simulink model "NXT_circle"  (R2024b)
settings: Solver=FixedStepDiscrete  StartTime=0.0  StopTime=inf  FixedStep=Ts  RelTol=1e-3
values from neighbouring files (symbols this model uses):
  dt = 0.005    [main.m]    (also in make_smooth.m)
  joint1_pos_circle = [0 joint1_pos_circle]    [generate_circle_trajectory.m]
  joint2_pos_circle = [0 joint2_pos_circle]    [generate_circle_trajectory.m]
  joint3_pos_circle = [0]    [generate_circle_trajectory.m]
  Kd = 2    [main.m]
  Kp = 25    [main.m]
  motor1_vel_circle = [0 motor1_vel_circle]    [generate_circle_trajectory.m]
  motor2_vel_circle = [0 motor2_vel_circle]    [generate_circle_trajectory.m]
  motor3_vel_circle = [0 motor3_vel_circle]    [generate_circle_trajectory.m]
  Ts_traj = 0.1    [main.m]
libraries: legonxtlib x6, cstblocks x3
settings Model: SimulationMode=external  ExtModeTrigDuration=2  Creator=pwterry
settings SolverCC: AlgebraicLoopSolver=TrustRegion
settings DataIOCC: LimitDataPoints=on  SaveFormat=Array  ReturnWorkspaceOutputs=off
settings OptimizationCC: LifeSpan=1  EfficientTunableParamExpr=on
settings DebuggingCC: UnderspecifiedInitializationDetection=Classic  MergeDetectMultiDrivingBlocksExec=none  UnconnectedInputMsg=warning  UnconnectedOutputMsg=warning  UnconnectedLineMsg=warning  SFUnexpectedBacktrackingDiag=warning  SFNoUnconditionalDefaultTransitionDiag=warning  SFExecutionAtInitializationDiag=none  ArithmeticOperatorsInVariantConditions=warning
settings HardwareCC: ProdBitPerPointer=32  ProdBitPerSizeT=32  ProdBitPerPtrDiffT=32  ProdLargestAtomicInteger=Long  ProdIntDivRoundTo=Undefined  ProdWordSize=32  ProdHWDeviceType=ARM Compatible->ARM 7
settings ModelReferenceCC: PropagateSignalLabelsOutOfModel=off
settings SFSimCC: SimUseLocalCustomCode=off  MATLABDynamicMemAlloc=off  CustomCodeUndefinedFunction=UseInterfaceOnly
settings RTWCC: Description=Run on Target Hardware  SystemTargetFile=realtime.tlc  GenerateMakefile=off  TemplateMakefile=realtime.tmf  RTWVerbose=off  RTWUseLocalCustomCode=off  GPUComputeCapability=3.5
settings CodeAppCC: StateflowObjectComments=on
settings STFCustomTargetCC: TargetLibSuffix=.a  GenerateSampleERTMain=on  ERTCustomFileBanners=on  SupportNonInlinedSFcns=off  RemoveResetFunc=on  SupportVariableSizeSignals=on  MATLABClassNameForMDSCustomization=Simulink.SoftwareTarget.ERTCustomization  SystemTargetFile=realtime.tlc
settings ERTTargetCC: MultiwordLength=2048  GenerateSampleERTMain=on  ParMdlRefBuildCompliant=off  CompOptLevelCompliant=off  ConcurrentExecutionCompliant=off  CombineOutputUpdateFcns=off  SupportContinuousTime=on  SupportVariableSizeSignals=on  ModelStepFunctionPrototypeControlCompliant=off  CPPClassGenCompliant=off  UseToolchainInfoCompliant=off  ExtMode=on  ExtModeTransport=2  ExtModeMexArgs=0 233 9600 30  InlinedParameterPlacement=Hierarchical  ERTSrcFileBannerTemplate=realtime_code_template.cgt  ERTHdrFileBannerTemplate=realtime_code_template.cgt  ERTDataSrcFileTemplate=realtime_code_template.cgt  ERTDataHdrFileTemplate=realtime_code_template.cgt  ERTCustomFileTemplate=realtime_file_process.tlc  ConvertIfToSwitch=off  SuppressUnreachableDefaultCases=off  DynamicArrayContainerType=coder::array
settings ConfigComp: CovMetricSettings=dw  CovSaveCumulativeToWorkspaceVar=on  CovSaveSingleToWorkspaceVar=on  CovExternalEMLEnable=off  CovSFcnEnable=off

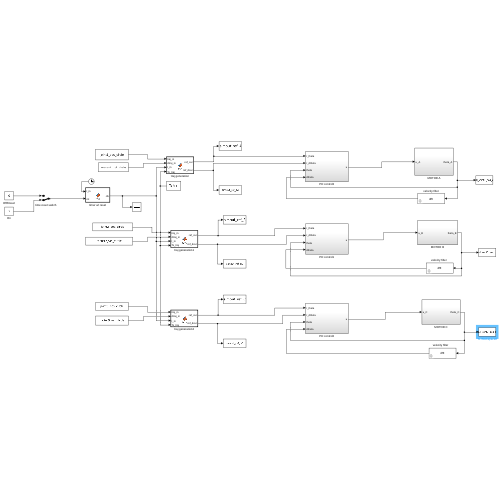
[thumbnail: Simulink's stored preview of the top-level diagram]
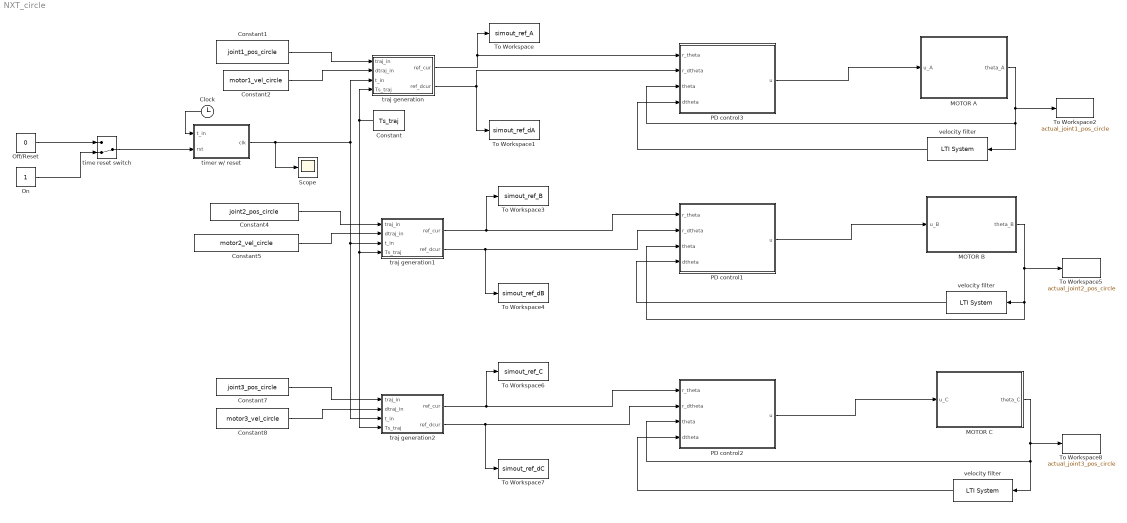
== system NXT_circle ==
  Clock : Clock
  Constant : Constant  Value=Ts_traj
  Constant1 : Constant  Value=joint1_pos_circle  SampleTime=dt
  Constant2 : Constant  Value=motor1_vel_circle  SampleTime=dt
  Constant4 : Constant  Value=joint2_pos_circle  SampleTime=dt
  Constant5 : Constant  Value=motor2_vel_circle  SampleTime=dt
  Constant7 : Constant  Value=joint3_pos_circle  SampleTime=dt
  Constant8 : Constant  Value=motor3_vel_circle  SampleTime=dt
  MOTOR A : Subsystem
  MOTOR B : Subsystem
  MOTOR C : Subsystem
  Off/Reset : Constant  Value=0
  On : Constant
  PD control1 : Subsystem
  PD control2 : Subsystem
  PD control3 : Subsystem
  Scope : Scope
  To Workspace : ToWorkspace  VariableName=simout_ref_A  SaveFormat=Structure With Time  SampleTime=-1
  To Workspace1 : ToWorkspace  VariableName=simout_ref_dA  SaveFormat=Structure With Time  SampleTime=-1
  To Workspace2 : ToWorkspace  VariableName=actual_joint1_pos_circle  SaveFormat=Structure With Time  SampleTime=dt
  To Workspace3 : ToWorkspace  VariableName=simout_ref_B  SaveFormat=Structure With Time  SampleTime=-1
  To Workspace4 : ToWorkspace  VariableName=simout_ref_dB  SaveFormat=Structure With Time  SampleTime=-1
  To Workspace5 : ToWorkspace  VariableName=actual_joint2_pos_circle  SaveFormat=Structure With Time  SampleTime=dt
  To Workspace6 : ToWorkspace  VariableName=simout_ref_C  SaveFormat=Structure With Time  SampleTime=-1
  To Workspace7 : ToWorkspace  VariableName=simout_ref_dC  SaveFormat=Structure With Time  SampleTime=-1
  To Workspace8 : ToWorkspace  VariableName=actual_joint3_pos_circle  SaveFormat=Structure With Time  SampleTime=dt
  time reset switch : ManualSwitch  CurrentSetting=0
  timer w/ reset : MATLAB Function  TreatAsAtomicUnit=on
  traj generation : MATLAB Function  TreatAsAtomicUnit=on
  traj generation1 : MATLAB Function  TreatAsAtomicUnit=on
  traj generation2 : MATLAB Function  TreatAsAtomicUnit=on
  velocity filter : cstblocks/LTI System  sys=dfft  IC=[]  PadeOrder=0
  "velocity filter  " : cstblocks/LTI System  sys=dfft  IC=[]  PadeOrder=0
  "velocity filter     " : cstblocks/LTI System  sys=dfft  IC=[]  PadeOrder=0
  wires:
  Constant/1 -> traj generation2/4(Ts_traj), traj generation1/4(Ts_traj), traj generation/4(Ts_traj)
  timer w/ reset/1(clk) -> Scope/1, traj generation1/3(t_in), traj generation2/3(t_in), traj generation/3(t_in)
  Constant1/1 -> traj generation/1(traj_in)
  Constant2/1 -> traj generation/2(dtraj_in)
  traj generation/1(ref_cur) -> PD control3/1(r_theta), To Workspace/1
  traj generation/2(ref_dcur) -> PD control3/2(r_dtheta), To Workspace1/1
  Constant4/1 -> traj generation1/1(traj_in)
  Constant5/1 -> traj generation1/2(dtraj_in)
  traj generation1/1(ref_cur) -> PD control1/1(r_theta), To Workspace3/1
  traj generation1/2(ref_dcur) -> PD control1/2(r_dtheta), To Workspace4/1
  Constant7/1 -> traj generation2/1(traj_in)
  Constant8/1 -> traj generation2/2(dtraj_in)
  traj generation2/1(ref_cur) -> PD control2/1(r_theta), To Workspace6/1
  traj generation2/2(ref_dcur) -> PD control2/2(r_dtheta), To Workspace7/1
  MOTOR A/1(theta_A) -> To Workspace2/1, PD control3/3(theta), velocity filter/1
  velocity filter/1 -> PD control3/4(dtheta)
  MOTOR B/1(theta_B) -> To Workspace5/1, PD control1/3(theta), "velocity filter  "/1
  "velocity filter  "/1 -> PD control1/4(dtheta)
  "velocity filter     "/1 -> PD control2/4(dtheta)
  MOTOR C/1(theta_C) -> To Workspace8/1, PD control2/3(theta), "velocity filter     "/1
  Off/Reset/1 -> time reset switch/1
  On/1 -> time reset switch/2
  time reset switch/1 -> timer w/ reset/2(rst)
  Clock/1 -> timer w/ reset/1(t_in)
  PD control3/1(u) -> MOTOR A/1(u_A)
  PD control1/1(u) -> MOTOR B/1(u_B)
  PD control2/1(u) -> MOTOR C/1(u_C)

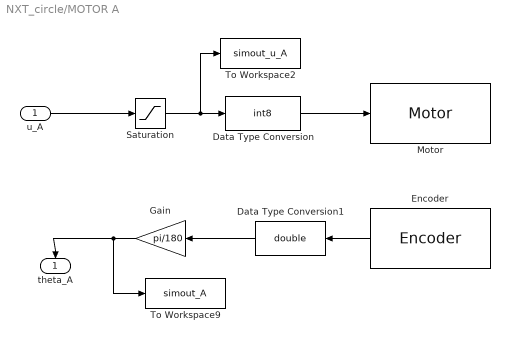
== system NXT_circle/MOTOR A ==
  u_A : Inport
  Data Type Conversion : DataTypeConversion  OutDataTypeStr=int8  SaturateOnIntegerOverflow=off  RndMeth=Floor
  Data Type Conversion1 : DataTypeConversion  OutDataTypeStr=double  SaturateOnIntegerOverflow=off  RndMeth=Floor
  Encoder : legonxtlib/Encoder  portNumber=A  opMode=No reset  sampleTime=Ts
  Gain : Gain  Gain=pi/180
  Motor : legonxtlib/Motor  sportNumber=A  sstopAction=Brake
  Saturation : Saturate  UpperLimit=100  LowerLimit=-100
  To Workspace2 : ToWorkspace  VariableName=simout_u_A  SaveFormat=Structure With Time  SampleTime=-1
  To Workspace9 : ToWorkspace  VariableName=simout_A  SaveFormat=Structure With Time  SampleTime=-1
  theta_A : Outport
  wires:
  u_A/1 -> Saturation/1
  Data Type Conversion1/1 -> Gain/1
  Saturation/1 -> To Workspace2/1, Data Type Conversion/1
  Encoder/1 -> Data Type Conversion1/1
  Data Type Conversion/1 -> Motor/1
  Gain/1 -> theta_A/1, To Workspace9/1

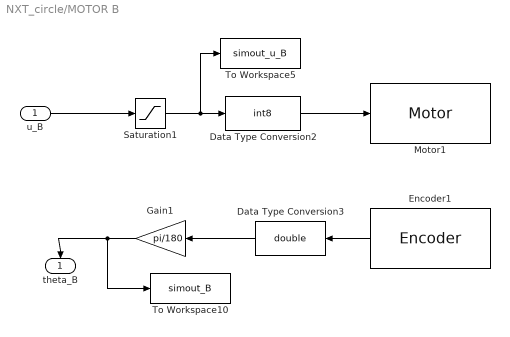
== system NXT_circle/MOTOR B ==
  u_B : Inport
  Data Type Conversion2 : DataTypeConversion  OutDataTypeStr=int8  SaturateOnIntegerOverflow=off  RndMeth=Floor
  Data Type Conversion3 : DataTypeConversion  OutDataTypeStr=double  SaturateOnIntegerOverflow=off  RndMeth=Floor
  Encoder1 : legonxtlib/Encoder  portNumber=B  opMode=No reset  sampleTime=Ts
  Gain1 : Gain  Gain=pi/180
  Motor1 : legonxtlib/Motor  sportNumber=B  sstopAction=Brake
  Saturation1 : Saturate  UpperLimit=100  LowerLimit=-100
  To Workspace10 : ToWorkspace  VariableName=simout_B  SaveFormat=Structure With Time  SampleTime=-1
  To Workspace5 : ToWorkspace  VariableName=simout_u_B  SaveFormat=Structure With Time  SampleTime=-1
  theta_B : Outport
  wires:
  Encoder1/1 -> Data Type Conversion3/1
  u_B/1 -> Saturation1/1
  Saturation1/1 -> To Workspace5/1, Data Type Conversion2/1
  Data Type Conversion3/1 -> Gain1/1
  Data Type Conversion2/1 -> Motor1/1
  Gain1/1 -> theta_B/1, To Workspace10/1

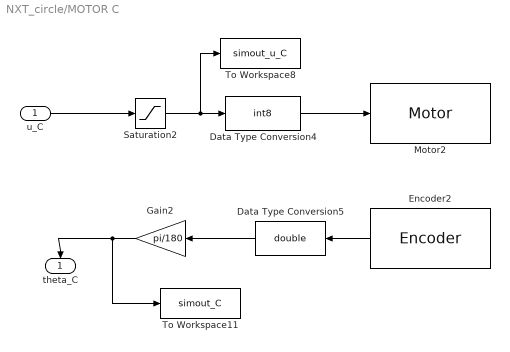
== system NXT_circle/MOTOR C ==
  u_C : Inport
  Data Type Conversion4 : DataTypeConversion  OutDataTypeStr=int8  SaturateOnIntegerOverflow=off  RndMeth=Floor
  Data Type Conversion5 : DataTypeConversion  OutDataTypeStr=double  SaturateOnIntegerOverflow=off  RndMeth=Floor
  Encoder2 : legonxtlib/Encoder  portNumber=C  opMode=No reset  sampleTime=Ts
  Gain2 : Gain  Gain=pi/180
  Motor2 : legonxtlib/Motor  sportNumber=C  sstopAction=Brake
  Saturation2 : Saturate  UpperLimit=100  LowerLimit=-100
  To Workspace11 : ToWorkspace  VariableName=simout_C  SaveFormat=Structure With Time  SampleTime=-1
  To Workspace8 : ToWorkspace  VariableName=simout_u_C  SaveFormat=Structure With Time  SampleTime=-1
  theta_C : Outport
  wires:
  Encoder2/1 -> Data Type Conversion5/1
  Data Type Conversion4/1 -> Motor2/1
  Data Type Conversion5/1 -> Gain2/1
  Gain2/1 -> theta_C/1, To Workspace11/1
  Saturation2/1 -> To Workspace8/1, Data Type Conversion4/1
  u_C/1 -> Saturation2/1

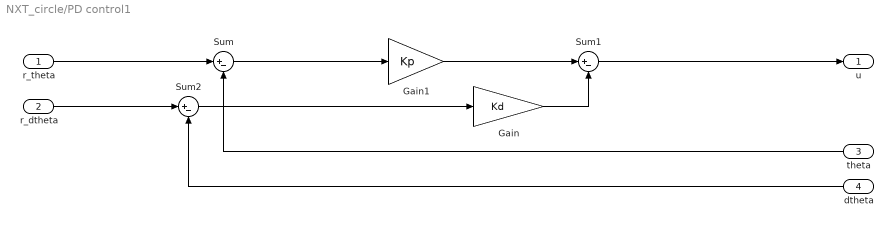
== system NXT_circle/PD control1 ==
  r_theta : Inport
  r_dtheta : Inport  Port=2
  theta : Inport  Port=3
  dtheta : Inport  Port=4
  Gain : Gain  Gain=Kd  SampleTime=dt
  Gain1 : Gain  Gain=Kp  SampleTime=dt
  Sum : Sum  Inputs=|+-
  Sum1 : Sum  Inputs=|+-
  Sum2 : Sum  Inputs=|+-
  u : Outport
  wires:
  r_theta/1 -> Sum/1
  Sum/1 -> Gain1/1
  theta/1 -> Sum/2
  dtheta/1 -> Sum2/2
  Gain1/1 -> Sum1/1
  Sum1/1 -> u/1
  r_dtheta/1 -> Sum2/1
  Sum2/1 -> Gain/1
  Gain/1 -> Sum1/2

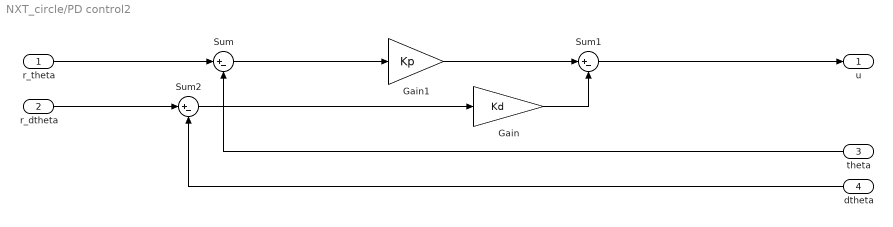
== system NXT_circle/PD control2 ==
  r_theta : Inport
  r_dtheta : Inport  Port=2
  theta : Inport  Port=3
  dtheta : Inport  Port=4
  Gain : Gain  Gain=Kd  SampleTime=dt
  Gain1 : Gain  Gain=Kp  SampleTime=dt
  Sum : Sum  Inputs=|+-
  Sum1 : Sum  Inputs=|+-
  Sum2 : Sum  Inputs=|+-
  u : Outport
  wires:
  r_theta/1 -> Sum/1
  Sum/1 -> Gain1/1
  theta/1 -> Sum/2
  dtheta/1 -> Sum2/2
  Gain1/1 -> Sum1/1
  Sum1/1 -> u/1
  r_dtheta/1 -> Sum2/1
  Sum2/1 -> Gain/1
  Gain/1 -> Sum1/2

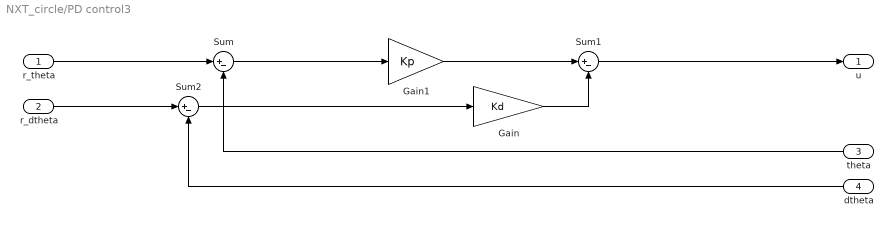
== system NXT_circle/PD control3 ==
  r_theta : Inport
  r_dtheta : Inport  Port=2
  theta : Inport  Port=3
  dtheta : Inport  Port=4
  Gain : Gain  Gain=Kd  SampleTime=dt
  Gain1 : Gain  Gain=Kp  SampleTime=dt
  Sum : Sum  Inputs=|+-
  Sum1 : Sum  Inputs=|+-
  Sum2 : Sum  Inputs=|+-
  u : Outport
  wires:
  r_theta/1 -> Sum/1
  Sum/1 -> Gain1/1
  theta/1 -> Sum/2
  dtheta/1 -> Sum2/2
  Gain1/1 -> Sum1/1
  Sum1/1 -> u/1
  r_dtheta/1 -> Sum2/1
  Sum2/1 -> Gain/1
  Gain/1 -> Sum1/2

== matlab function NXT_circle/traj generation1 ==
  data: traj_in input; dtraj_in input; ref_cur output; t_in input; Ts_traj input; ref_dcur output
function [ref_cur, ref_dcur] = fcn(traj_in, dtraj_in, t_in, Ts_traj)
t_offset = 1;   %amt of seconds to wait before starting traj

base_numPts_per_sec = length(traj_in)/(Ts_traj*length(traj_in));
scaleFactor = 1; %Time scaling factor (# of trajectory points per second multiplier)
%Tweaking this will speed-up or slow-down the playback of traj, allowing
%for some control over resolution.
scaling = scaleFactor*base_numPts_per_sec; 
t_cur = t_in-t_offset;
time = max(t_cur,0);
%Compute the current index in the trajectory array
index_fraction = scaling*time + 1;
index = floor(index_fraction);
frac_add = index_fraction - index; % additional amount "beyond" index
%Extract the current position from the trajectory (plus interp)
if (index < length(traj_in))
    
    theta_out = (1-frac_add)*double(traj_in(index)) + ...
        frac_add*double(traj_in(index+1));
    
    dtheta_out = (1-frac_add)*double(dtraj_in(index)) + ...
        frac_add*double(dtraj_in(index+1));
    
else %If we run out of data, continue outputting the last value
    theta_out = double(traj_in(length(traj_in)));
    dtheta_out = double(dtraj_in(length(dtraj_in)));
end
ref_cur = theta_out;
ref_dcur = dtheta_out;




end

== matlab function NXT_circle/traj generation2 ==
  data: traj_in input; dtraj_in input; ref_cur output; t_in input; Ts_traj input; ref_dcur output
function [ref_cur, ref_dcur] = fcn(traj_in, dtraj_in, t_in, Ts_traj)
t_offset = 1;   %amt of seconds to wait before starting traj

base_numPts_per_sec = length(traj_in)/(Ts_traj*length(traj_in));
scaleFactor = 1; %Time scaling factor (# of trajectory points per second multiplier)
%Tweaking this will speed-up or slow-down the playback of traj, allowing
%for some control over resolution.
scaling = scaleFactor*base_numPts_per_sec; 
t_cur = t_in-t_offset;
time = max(t_cur,0);
%Compute the current index in the trajectory array
index_fraction = scaling*time + 1;
index = floor(index_fraction);
frac_add = index_fraction - index; % additional amount "beyond" index
%Extract the current position from the trajectory (plus interp)
if (index < length(traj_in))
    
    theta_out = (1-frac_add)*double(traj_in(index)) + ...
        frac_add*double(traj_in(index+1));
    
    dtheta_out = (1-frac_add)*double(dtraj_in(index)) + ...
        frac_add*double(dtraj_in(index+1));
    
else %If we run out of data, continue outputting the last value
    theta_out = double(traj_in(length(traj_in)));
    dtheta_out = double(dtraj_in(length(dtraj_in)));
end
ref_cur = theta_out;
ref_dcur = dtheta_out;




end

== matlab function NXT_circle/timer w// reset ==
  data: t_in input; clk output; rst input
function clk = fcn(t_in, rst)
persistent t_off last_rst
if isempty(t_off)
    t_off = 0;
end
if isempty(last_rst)
    last_rst = 0;
end

%if rest switch was pressed, use current time as t_offset
if abs(rst - last_rst) ~= 0
   t_off = t_in;    
end

if rst == 0
    clk = 0;    %force time to wait if reset is on
else
    clk = t_in - t_off; %output clock
end
last_rst = rst;     %update reset var

== matlab function NXT_circle/traj generation ==
  data: traj_in input; dtraj_in input; ref_cur output; t_in input; Ts_traj input; ref_dcur output
function [ref_cur, ref_dcur] = fcn(traj_in, dtraj_in, t_in, Ts_traj)
t_offset = 1;   %amt of seconds to wait before starting traj

base_numPts_per_sec = length(traj_in)/(Ts_traj*length(traj_in));
scaleFactor = 1; %Time scaling factor (# of trajectory points per second multiplier)
%Tweaking this will speed-up or slow-down the playback of traj, allowing
%for some control over resolution.
scaling = scaleFactor*base_numPts_per_sec; 
t_cur = t_in-t_offset;
time = max(t_cur,0);
%Compute the current index in the trajectory array
index_fraction = scaling*time + 1;
index = floor(index_fraction);
frac_add = index_fraction - index; % additional amount "beyond" index
%Extract the current position from the trajectory (plus interp)
if (index < length(traj_in))
    
    theta_out = (1-frac_add)*double(traj_in(index)) + ...
        frac_add*double(traj_in(index+1));
    
    dtheta_out = (1-frac_add)*double(dtraj_in(index)) + ...
        frac_add*double(dtraj_in(index+1));
    
else %If we run out of data, continue outputting the last value
    theta_out = double(traj_in(length(traj_in)));
    dtheta_out = double(dtraj_in(length(dtraj_in)));
end
ref_cur = theta_out;
ref_dcur = dtheta_out;




end
